simulink model "turbine"  (R2015b)
settings: Solver=FixedStepDiscrete  StartTime=0.0  StopTime=10.0  RelTol=1e-3
undefined symbols (not defined in the file or in its folder): BSRmax, cp_exh, etaTmax, etaTmin, gamma_exh, k0, k1, Nt, p03, PiT, rTurb, T03
settings Model: Creator=fahle  LastModifiedBy=fahle

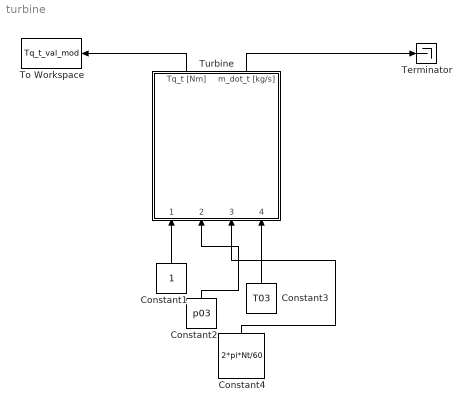
== system turbine ==
  Constant1 : Constant
  Constant2 : Constant  Value=p03
  Constant3 : Constant  Value=T03
  Constant4 : Constant  Value=2*pi*Nt/60
  Terminator : Terminator
  To Workspace : ToWorkspace  VariableName=Tq_t_val_mod  SampleTime=-1
  Turbine : Subsystem
  wires:
  Constant1/1 -> Turbine/1("p_t [Pa] ")
  Constant2/1 -> Turbine/2(p_em [Pa])
  Constant4/1 -> Turbine/3(w_tc [rad/s])
  Constant3/1 -> Turbine/4(T_em [k])
  Turbine/2(m_dot_t [kg/s]) -> Terminator/1
  Turbine/1(Tq_t [Nm]) -> To Workspace/1

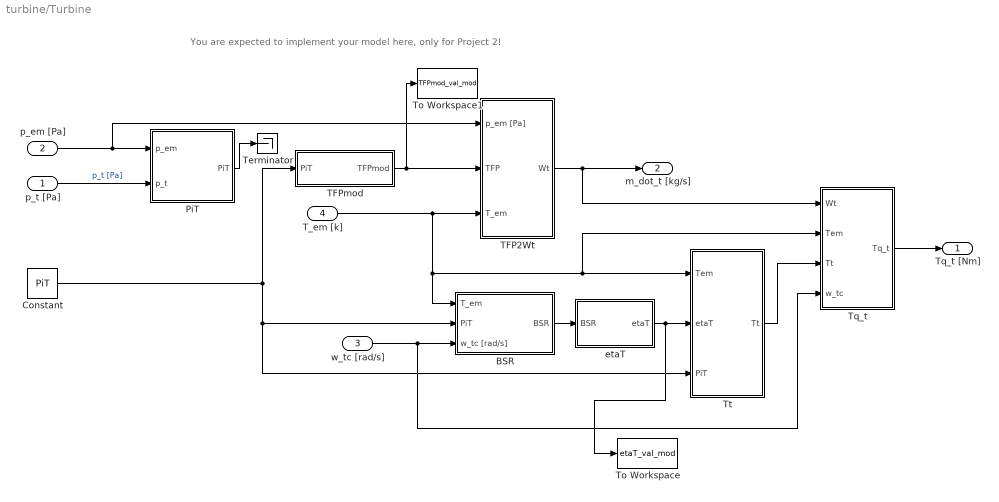
== system turbine/Turbine ==
  note: You are expected to implement your model here, only for Project 2!
  "p_t [Pa] " : Inport
  p_em [Pa] : Inport  Port=2
  w_tc [rad/s] : Inport  Port=3
  T_em [k] : Inport  Port=4
  BSR : Subsystem
  Constant : Constant  Value=PiT
  PiT : Subsystem
  TFP2Wt : Subsystem
  TFPmod : Subsystem
  Terminator : Terminator
  To Workspace : ToWorkspace  VariableName=etaT_val_mod  SampleTime=-1
  To Workspace1 : ToWorkspace  VariableName=TFPmod_val_mod  SampleTime=-1
  Tq_t : Subsystem
  Tt : Subsystem
  etaT : Subsystem
  Tq_t [Nm] : Outport
  m_dot_t [kg/s] : Outport  Port=2
  wires:
  Tq_t/1(Tq_t) -> Tq_t [Nm]/1
  Tt/1(Tt) -> Tq_t/3(Tt)
  etaT/1(etaT) -> To Workspace/1, Tt/2(etaT)
  T_em [k]/1 -> Tt/1(Tem), Tq_t/2(Tem), BSR/1(T_em), TFP2Wt/3(T_em)
  BSR/1(BSR) -> etaT/1(BSR)
  TFP2Wt/1(Wt) -> Tq_t/1(Wt), m_dot_t [kg/s]/1
  TFPmod/1(TFPmod) -> To Workspace1/1, TFP2Wt/2(TFP)
  Constant/1 -> TFPmod/1(PiT), Tt/3(PiT), BSR/2(PiT)
  p_em [Pa]/1 -> TFP2Wt/1(p_em [Pa]), PiT/1(p_em)
  "p_t [Pa] "/1 -> PiT/2(p_t)  "p_t [Pa]"
  w_tc [rad/s]/1 -> Tq_t/4(w_tc), BSR/3(w_tc [rad/s])
  PiT/1(PiT) -> Terminator/1

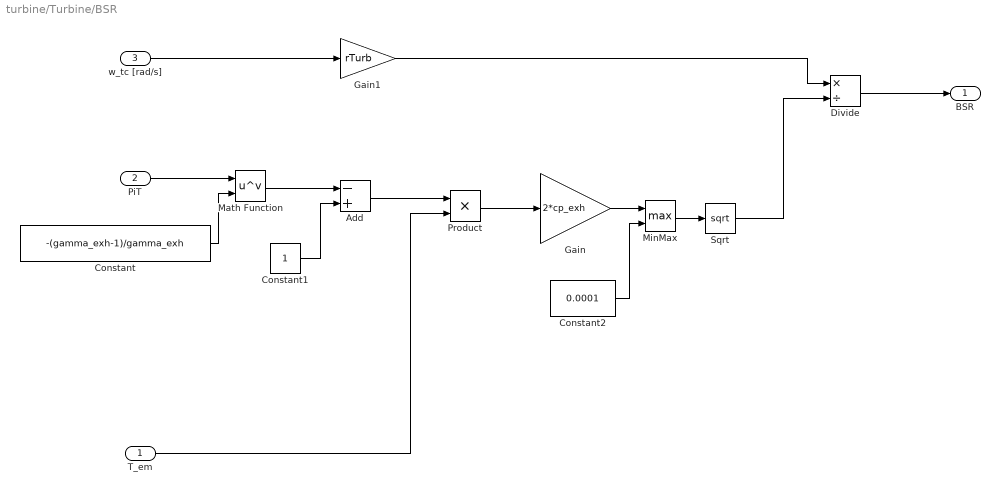
== system turbine/Turbine/BSR ==
  T_em : Inport
  PiT : Inport  Port=2
  w_tc [rad/s] : Inport  Port=3
  Add : Sum  Inputs=-+
  Constant : Constant  Value=-(gamma_exh-1)/gamma_exh
  Constant1 : Constant
  Constant2 : Constant  Value=0.0001
  Divide : Product  Inputs=*/
  Gain : Gain  Gain=2*cp_exh
  Gain1 : Gain  Gain=rTurb
  Math Function : Math  Operator=pow  SaturateOnIntegerOverflow=on
  MinMax : MinMax  Function=max  Inputs=2
  Product : Product
  Sqrt : Sqrt  SaturateOnIntegerOverflow=on
  BSR : Outport
  wires:
  PiT/1 -> Math Function/1
  Constant/1 -> Math Function/2
  Math Function/1 -> Add/1
  Constant1/1 -> Add/2
  Add/1 -> Product/1
  T_em/1 -> Product/2
  Product/1 -> Gain/1
  Constant2/1 -> MinMax/2
  Gain/1 -> MinMax/1
  MinMax/1 -> Sqrt/1
  Sqrt/1 -> Divide/2
  Gain1/1 -> Divide/1
  w_tc [rad/s]/1 -> Gain1/1
  Divide/1 -> BSR/1

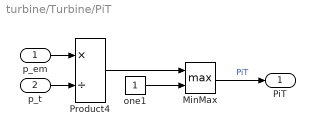
== system turbine/Turbine/PiT ==
  p_em : Inport
  p_t : Inport  Port=2
  MinMax : MinMax  Function=max  Inputs=2
  Product4 : Product  Inputs=*/  RndMeth=Zero
  one1 : Constant
  PiT : Outport
  wires:
  p_t/1 -> Product4/2
  MinMax/1 -> PiT/1  "PiT"
  p_em/1 -> Product4/1
  one1/1 -> MinMax/2
  Product4/1 -> MinMax/1

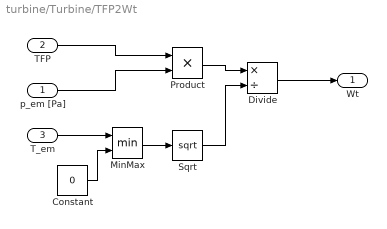
== system turbine/Turbine/TFP2Wt ==
  p_em [Pa] : Inport
  TFP : Inport  Port=2
  T_em : Inport  Port=3
  Constant : Constant  Value=0
  Divide : Product  Inputs=*/
  MinMax : MinMax  Inputs=2
  Product : Product
  Sqrt : Sqrt  SaturateOnIntegerOverflow=on
  Wt : Outport
  wires:
  Divide/1 -> Wt/1
  TFP/1 -> Product/1
  p_em [Pa]/1 -> Product/2
  Product/1 -> Divide/1
  Constant/1 -> MinMax/2
  T_em/1 -> MinMax/1
  MinMax/1 -> Sqrt/1
  Sqrt/1 -> Divide/2

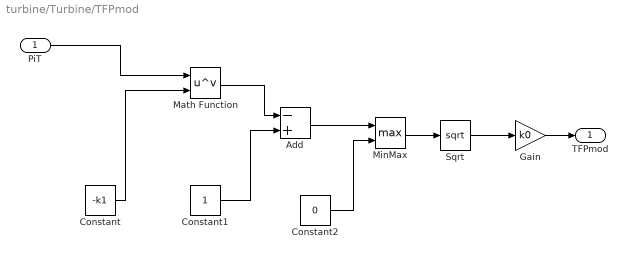
== system turbine/Turbine/TFPmod ==
  PiT : Inport
  Add : Sum  Inputs=-+
  Constant : Constant  Value=-k1
  Constant1 : Constant
  Constant2 : Constant  Value=0
  Gain : Gain  Gain=k0
  Math Function : Math  Operator=pow  SaturateOnIntegerOverflow=on
  MinMax : MinMax  Function=max  Inputs=2
  Sqrt : Sqrt  SaturateOnIntegerOverflow=on
  TFPmod : Outport
  wires:
  PiT/1 -> Math Function/1
  Constant/1 -> Math Function/2
  Math Function/1 -> Add/1
  Constant1/1 -> Add/2
  Constant2/1 -> MinMax/2
  Add/1 -> MinMax/1
  MinMax/1 -> Sqrt/1
  Sqrt/1 -> Gain/1
  Gain/1 -> TFPmod/1

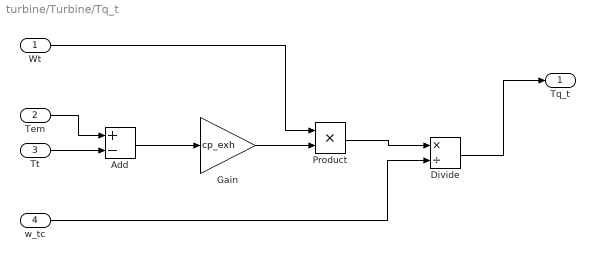
== system turbine/Turbine/Tq_t ==
  Wt : Inport
  Tem : Inport  Port=2
  Tt : Inport  Port=3
  w_tc : Inport  Port=4
  Add : Sum  Inputs=+-
  Divide : Product  Inputs=*/
  Gain : Gain  Gain=cp_exh
  Product : Product
  Tq_t : Outport
  wires:
  Tt/1 -> Add/2
  Tem/1 -> Add/1
  Add/1 -> Gain/1
  Gain/1 -> Product/2
  Wt/1 -> Product/1
  w_tc/1 -> Divide/2
  Product/1 -> Divide/1
  Divide/1 -> Tq_t/1

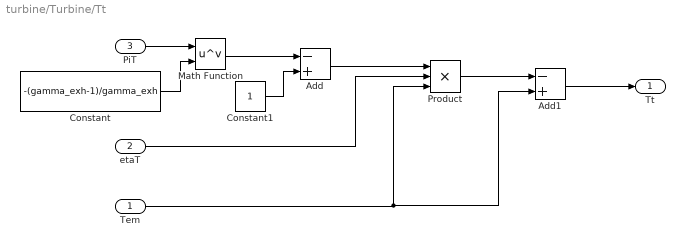
== system turbine/Turbine/Tt ==
  Tem : Inport
  etaT : Inport  Port=2
  PiT : Inport  Port=3
  Add : Sum  Inputs=-+
  Add1 : Sum  Inputs=-+
  Constant : Constant  Value=-(gamma_exh-1)/gamma_exh
  Constant1 : Constant
  Math Function : Math  Operator=pow  SaturateOnIntegerOverflow=on
  Product : Product  Inputs=3
  Tt : Outport
  wires:
  PiT/1 -> Math Function/1
  Constant/1 -> Math Function/2
  Math Function/1 -> Add/1
  Constant1/1 -> Add/2
  Add/1 -> Product/1
  etaT/1 -> Product/2
  Tem/1 -> Add1/2, Product/3
  Product/1 -> Add1/1
  Add1/1 -> Tt/1

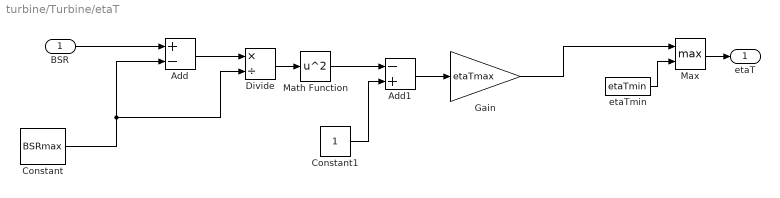
== system turbine/Turbine/etaT ==
  BSR : Inport
  Add : Sum  Inputs=+-
  Add1 : Sum  Inputs=-+
  Constant : Constant  Value=BSRmax
  Constant1 : Constant
  Divide : Product  Inputs=*/
  Gain : Gain  Gain=etaTmax
  Math Function : Math  Operator=square  SaturateOnIntegerOverflow=on
  Max : MinMax  Function=max  Inputs=2
  etaTmin : Constant  Value=etaTmin
  etaT : Outport
  wires:
  etaTmin/1 -> Max/2
  Max/1 -> etaT/1
  BSR/1 -> Add/1
  Constant/1 -> Divide/2, Add/2
  Add/1 -> Divide/1
  Divide/1 -> Math Function/1
  Math Function/1 -> Add1/1
  Constant1/1 -> Add1/2
  Add1/1 -> Gain/1
  Gain/1 -> Max/1
